simulink model "slosh_separated_architecture"  (R2025b)
settings: Solver=ode45  StartTime=0.0  StopTime=20  RelTol=1e-3
settings Model: Creator=piepe  LastModifiedBy=piepe

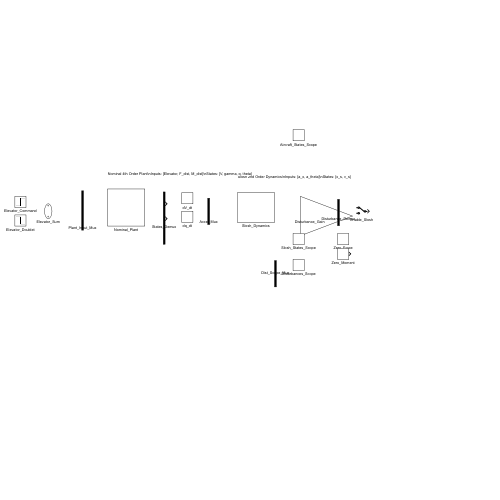
[thumbnail: Simulink's stored preview of the top-level diagram]
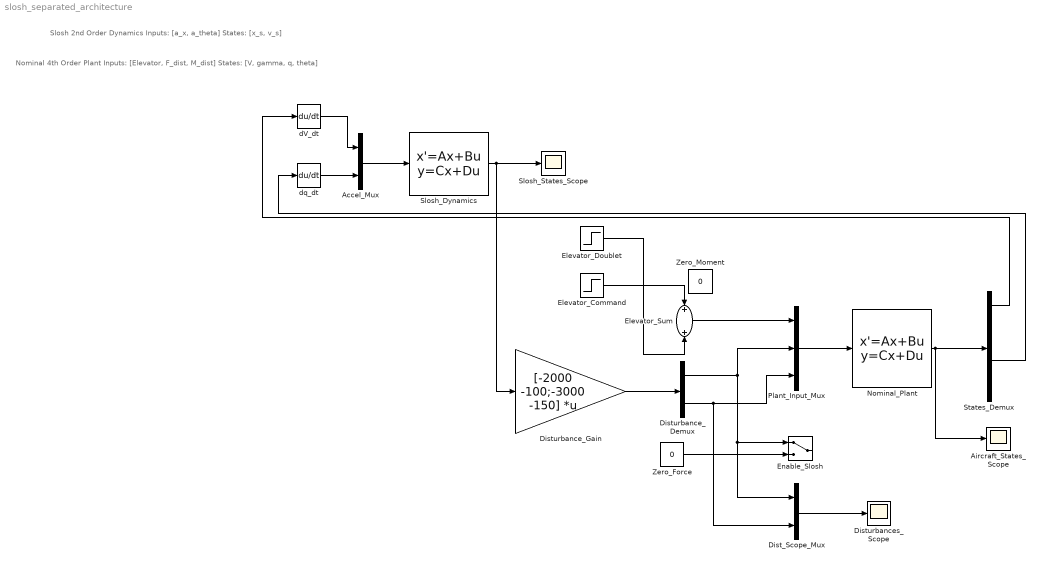
== system slosh_separated_architecture ==
  note: Nominal 4th Order Plant\nInputs: [Elevator, F_dist, M_dist]\nStates: [V, gamma, q, theta]
  note: Slosh 2nd Order Dynamics\nInputs: [a_x, a_theta]\nStates: [x_s, v_s]
  Accel_Mux : Mux  Inputs=2
  Aircraft_States_Scope : Scope
  Dist_Scope_Mux : Mux  Inputs=2
  Disturbance_Demux : Demux  Outputs=2
  Disturbance_Gain : Gain  Gain=[-2000 -100;-3000 -150]  Multiplication=Matrix(K*u)
  Disturbances_Scope : Scope
  Elevator_Command : Step  Time=2  After=0.1  SampleTime=0
  Elevator_Doublet : Step  Time=3  After=-0.1  SampleTime=0
  Elevator_Sum : Sum
  Enable_Slosh : ManualSwitch
  Nominal_Plant : StateSpace  A=[-0.05 -9.81 0 0;-0.01 0 1 0;0 -0.000327 -0.000133333333333333 0;0 0 1 0]  B=[0.0002 0.0002 0;0 0 0;-0.000333333333333333 0 6.66666666666667e-05;0 0 0]  C=[1 0 0 0;0 1 0 0;0 0 1 0;0 0 0 1]  D=[0 0 0;0 0 0;0 0 0;0 0 0]  InitialCondition=[0;0.05;0;0.05]
  Plant_Input_Mux : Mux  Inputs=3
  Slosh_Dynamics : StateSpace  A=[0 1;-4 -0.2]  B=[0 0;1 1.5]  C=[1 0;0 1]  D=[0 0;0 0]  InitialCondition=[0.1;0]
  Slosh_States_Scope : Scope
  States_Demux : Demux
  Zero_Force : Constant  Value=0
  Zero_Moment : Constant  Value=0
  dV_dt : Derivative
  dq_dt : Derivative
  wires:
  dq_dt/1 -> Accel_Mux/2
  dV_dt/1 -> Accel_Mux/1
  Disturbance_Gain/1 -> Disturbance_Demux/1
  Slosh_Dynamics/1 -> Disturbance_Gain/1, Slosh_States_Scope/1
  Accel_Mux/1 -> Slosh_Dynamics/1
  Elevator_Command/1 -> Elevator_Sum/1
  Elevator_Doublet/1 -> Elevator_Sum/2
  Elevator_Sum/1 -> Plant_Input_Mux/1
  Disturbance_Demux/1 -> Dist_Scope_Mux/1, Enable_Slosh/1, Plant_Input_Mux/2
  Plant_Input_Mux/1 -> Nominal_Plant/1
  Disturbance_Demux/2 -> Dist_Scope_Mux/2, Plant_Input_Mux/3
  Dist_Scope_Mux/1 -> Disturbances_Scope/1
  Zero_Force/1 -> Enable_Slosh/2
  States_Demux/1 -> dV_dt/1
  Nominal_Plant/1 -> States_Demux/1, Aircraft_States_Scope/1
  States_Demux/3 -> dq_dt/1
